simulink model "cobot_dy_create_model"  (R2015b)
settings: Solver=FixedStepAuto  StartTime=0.0  StopTime=10  FixedStep=0.01  RelTol=1e-3
values from neighbouring files (symbols this model uses):
  g = 9.8065    [cobot_gen_traj_and_mass_param.m]    (also in ts2.m; ts3.m)
  ic1 = [ic1xx -ic1xy -ic1xz ... (first row only)    [cobot_gen_traj_and_mass_param.m]
  ic2 = [ic2xx -ic2xy -ic2xz ... (first row only)    [cobot_gen_traj_and_mass_param.m]
  ic3 = [ic3xx -ic3xy -ic3xz ... (first row only)    [cobot_gen_traj_and_mass_param.m]
  ic4 = [ic4xx -ic4xy -ic4xz ... (first row only)    [cobot_gen_traj_and_mass_param.m]
  ic5 = [ic5xx -ic5xy -ic5xz ... (first row only)    [cobot_gen_traj_and_mass_param.m]
  ic6 = [ic6xx -ic6xy -ic6xz ... (first row only)    [cobot_gen_traj_and_mass_param.m]
  m1 = 4.43412756    [cobot_gen_traj_and_mass_param.m]
  m2 = 16.84660904    [cobot_gen_traj_and_mass_param.m]
  m3 = 4.60251258    [cobot_gen_traj_and_mass_param.m]
  m4 = 0.47079045    [cobot_gen_traj_and_mass_param.m]
  m5 = 0.07740646    [cobot_gen_traj_and_mass_param.m]
  m6 = 0.00343612    [cobot_gen_traj_and_mass_param.m]
  P001 = [0 0 d1]'    [cobot_gen_traj_and_mass_param.m]
  P223 = [a3 0 0]'    [cobot_gen_traj_and_mass_param.m]
  P334 = [a4 0 d4]'    [cobot_gen_traj_and_mass_param.m]
  P445 = [0 d5 0]'    [cobot_gen_traj_and_mass_param.m]
  P556 = [0 -d6 0]'    [cobot_gen_traj_and_mass_param.m]
  P667 = [0 0 0]'    [cobot_gen_traj_and_mass_param.m]
  Pc111 = [pc1x pc1y pc1z]'    [cobot_gen_traj_and_mass_param.m]
  Pc222 = [pc2x pc2y pc2z]'    [cobot_gen_traj_and_mass_param.m]
  Pc333 = [pc3x pc3y pc3z]'    [cobot_gen_traj_and_mass_param.m]
  Pc444 = [pc4x pc4y pc4z]'    [cobot_gen_traj_and_mass_param.m]
  Pc555 = [pc5x pc5y pc5z]'    [cobot_gen_traj_and_mass_param.m]
  Pc666 = [pc6x pc6y pc6z]'    [cobot_gen_traj_and_mass_param.m]
libraries: mblibv1 x29
settings Model: Creator=user  LastModifiedBy=12157
settings ConfigComp: CovHTMLOptions=-sRT=1 -sVT=0 -aTS=1 -bRG=1 -bTC=1 -hTR=0 -nFC=0 -nFD=1 -scm=1 -bcm=1 -xEv=0 -xEM=0
settings SimMechanicsCC: VisOnUpdateDiagram=on  VisDuringSimulation=on  LastVizWinPosition=[1 41 1920 938]  CamPosition=[6.48278;4.07346;8.12681;]  CamTarget=[-0.751108;-0.0621973;-0.55549;]  CamUpVector=[-0.477891;-0.569017;0.669208;]  CamHeight=1.40512  VisBackgroundColor=[0.9;0.9;0.95;]  DefaultBodyColor=[1;0;0;]

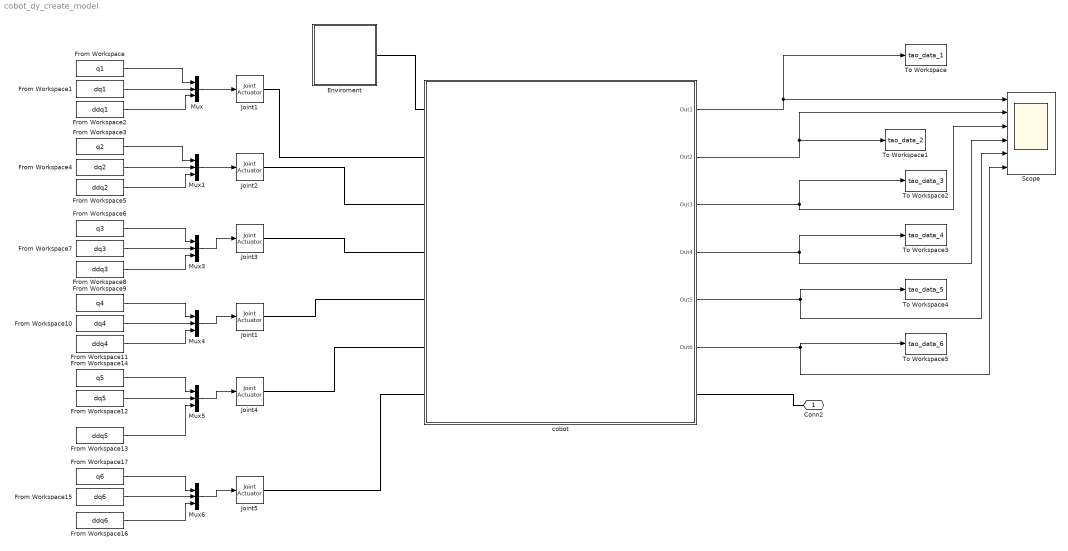
== system cobot_dy_create_model ==
  Enviroment : Subsystem
  From Workspace : FromWorkspace  VariableName=q1  SampleTime=0.01
  From Workspace1 : FromWorkspace  VariableName=dq1  SampleTime=0.01
  From Workspace10 : FromWorkspace  VariableName=dq4  SampleTime=0.01
  From Workspace11 : FromWorkspace  VariableName=ddq4  SampleTime=0.01
  From Workspace12 : FromWorkspace  VariableName=dq5  SampleTime=0.01
  From Workspace13 : FromWorkspace  VariableName=ddq5  SampleTime=0.01
  From Workspace14 : FromWorkspace  VariableName=q5  SampleTime=0.01
  From Workspace15 : FromWorkspace  VariableName=dq6  SampleTime=0.01
  From Workspace16 : FromWorkspace  VariableName=ddq6  SampleTime=0.01
  From Workspace17 : FromWorkspace  VariableName=q6  SampleTime=0.01
  From Workspace2 : FromWorkspace  VariableName=ddq1  SampleTime=0.01
  From Workspace3 : FromWorkspace  VariableName=q2  SampleTime=0.01
  From Workspace4 : FromWorkspace  VariableName=dq2  SampleTime=0.01
  From Workspace5 : FromWorkspace  VariableName=ddq2  SampleTime=0.01
  From Workspace6 : FromWorkspace  VariableName=q3  SampleTime=0.01
  From Workspace7 : FromWorkspace  VariableName=dq3  SampleTime=0.01
  From Workspace8 : FromWorkspace  VariableName=ddq3  SampleTime=0.01
  From Workspace9 : FromWorkspace  VariableName=q4  SampleTime=0.01
  Joint{1,3..5} (4 alike) : mblibv1/Sensors &  Actuators/Joint Actuator  UpdateFromCAD=off  PhysicalDomain=Mechanical  PortType=blob  ActuationStyle=Motion  AngleUnits=deg  ArcVelocityUnits=deg/s  ArcAccelerationUnits=deg/s^2  CoordPositionUnits=m  VelocityUnits=m/s  AccelerationUnits=m/s^2  ForceUnits=N  TorqueUnits=N*m  ActiveIO=on  Width=3  DialogClass=MechanicalActuatorBlock  Primitive=R1  ReferenceFrame=Absolute (World)
  "Joint1 " : mblibv1/Sensors &  Actuators/Joint Actuator  UpdateFromCAD=off  PhysicalDomain=Mechanical  PortType=blob  ActuationStyle=Motion  AngleUnits=deg  ArcVelocityUnits=deg/s  ArcAccelerationUnits=deg/s^2  CoordPositionUnits=m  VelocityUnits=m/s  AccelerationUnits=m/s^2  ForceUnits=N  TorqueUnits=N*m  ActiveIO=on  Width=3  DialogClass=MechanicalActuatorBlock  Primitive=R1  ReferenceFrame=Absolute (World)
  "Joint2 " : mblibv1/Sensors &  Actuators/Joint Actuator  UpdateFromCAD=off  PhysicalDomain=Mechanical  PortType=blob  ActuationStyle=Motion  AngleUnits=deg  ArcVelocityUnits=deg/s  ArcAccelerationUnits=deg/s^2  CoordPositionUnits=m  VelocityUnits=m/s  AccelerationUnits=m/s^2  ForceUnits=N  TorqueUnits=N*m  ActiveIO=on  Width=3  DialogClass=MechanicalActuatorBlock  Primitive=R1  ReferenceFrame=Absolute (World)
  Mux{,1,3..6} (6 alike) : Mux  Inputs=3
  Scope : Scope  NumInputPorts=6
  To Workspace : ToWorkspace  VariableName=tao_data_1  SaveFormat=Timeseries  SampleTime=-1
  To Workspace1 : ToWorkspace  VariableName=tao_data_2  SaveFormat=Timeseries  SampleTime=-1
  To Workspace2 : ToWorkspace  VariableName=tao_data_3  SaveFormat=Timeseries  SampleTime=-1
  To Workspace3 : ToWorkspace  VariableName=tao_data_4  SaveFormat=Timeseries  SampleTime=-1
  To Workspace4 : ToWorkspace  VariableName=tao_data_5  SaveFormat=Timeseries  SampleTime=-1
  To Workspace5 : ToWorkspace  VariableName=tao_data_6  SaveFormat=Timeseries  SampleTime=-1
  cobot : Subsystem
      mask Display: image('cobot.png')
  Conn2 : PMIOPort  Port=1  Side=Left
  wires:
  From Workspace/1 -> Mux/1
  From Workspace1/1 -> Mux/2
  From Workspace2/1 -> Mux/3
  Mux/1 -> "Joint1 "/1
  From Workspace3/1 -> Mux1/1
  From Workspace4/1 -> Mux1/2
  From Workspace5/1 -> Mux1/3
  Mux1/1 -> "Joint2 "/1
  From Workspace6/1 -> Mux3/1
  From Workspace7/1 -> Mux3/2
  From Workspace8/1 -> Mux3/3
  Mux3/1 -> Joint3/1
  From Workspace9/1 -> Mux4/1
  From Workspace10/1 -> Mux4/2
  From Workspace11/1 -> Mux4/3
  Mux4/1 -> Joint1/1
  From Workspace14/1 -> Mux5/1
  From Workspace12/1 -> Mux5/2
  From Workspace13/1 -> Mux5/3
  Mux5/1 -> Joint4/1
  From Workspace17/1 -> Mux6/1
  From Workspace15/1 -> Mux6/2
  From Workspace16/1 -> Mux6/3
  Mux6/1 -> Joint5/1
  cobot/2(Out2) -> Scope/2, To Workspace1/1
  cobot/3(Out3) -> To Workspace2/1, Scope/3
  cobot/4(Out4) -> To Workspace3/1, Scope/4
  cobot/5(Out5) -> Scope/5, To Workspace4/1
  cobot/6(Out6) -> Scope/6, To Workspace5/1
  cobot/1(Out1) -> To Workspace/1, Scope/1
  connections:
  "Joint1 "/RConn1 -- cobot/LConn2
  Conn2/RConn1 -- cobot/RConn1
  Enviroment/RConn1 -- cobot/LConn1
  "Joint2 "/RConn1 -- cobot/LConn3
  Joint3/RConn1 -- cobot/LConn4
  Joint1/RConn1 -- cobot/LConn5
  Joint4/RConn1 -- cobot/LConn6
  Joint5/RConn1 -- cobot/LConn7

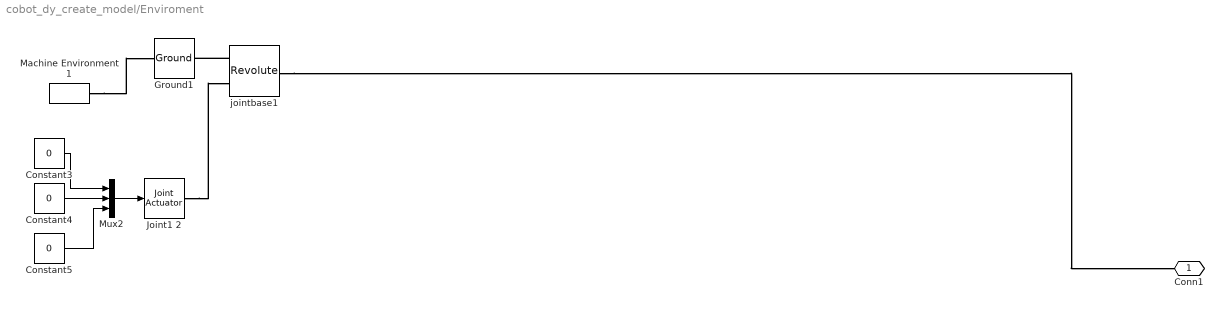
== system cobot_dy_create_model/Enviroment ==
  Constant3 : Constant  Value=0
  Constant4 : Constant  Value=0
  Constant5 : Constant  Value=0
  Ground1 : mblibv1/Bodies/Ground  UpdateFromCAD=off  LeftPortType=env  RightPortType=workingframe  PhysicalDomain=Mechanical  DialogClass=GroundBlock  CoordPosition=[0 0 0]  CoordPositionUnits=m  StateVectorMgrId=0  MachineId=[1 0]  ShowEnvPort=on  ParameterChecksum=[103943624, 4286749661, 2266336483, 2778931322]  TopologyChecksum=[1185680921, 963316717, 888619321, 413900908]
  Joint1 2 : mblibv1/Sensors &  Actuators/Joint Actuator  UpdateFromCAD=off  PhysicalDomain=Mechanical  PortType=blob  ActuationStyle=Motion  AngleUnits=deg  ArcVelocityUnits=deg/s  ArcAccelerationUnits=deg/s^2  CoordPositionUnits=m  VelocityUnits=m/s  AccelerationUnits=m/s^2  ForceUnits=N  TorqueUnits=N*m  ActiveIO=on  Width=3  DialogClass=MechanicalActuatorBlock  Primitive=R1  ReferenceFrame=Absolute (World)
  Machine Environment1 : mblibv1/Bodies/Machine Environment  PortType=env  PhysicalDomain=Mechanical  DialogTemplateClass=MECH.MachineEnvironment  SyncWhenCopied=off  Gravity=[0 0 -g]  GravityUnits=m/s^2  GravityAsSignal=off  Dimensionality=Auto-detect  AnalysisType=Forward dynamics  LinearAssemblyTolerance=1e-3  LinearAssemblyToleranceUnits=m  AngularAssemblyTolerance=1e-3  AngularAssemblyToleranceUnits=rad  ConstraintSolverType=Stabilizing  ConstraintRelTolerance=1e-4  ConstraintAbsTolerance=1e-4  UseRobustSingularityHandling=off  RedundancyAnalysisToleranceType=Automatically select tolerance  RedundancyAnalysisTolerance=1e-14  StatePerturbationType=Fixed  PerturbationSize=1e-5  VisualizeMachine=on  BodyVisualizationType=Use model default body geometries  BodyColorSelMode=Use model default  DefaultBodyColor=[1 0 0]
  Mux2 : Mux  Inputs=3
  jointbase1 : mblibv1/Joints/Revolute  LConnTagsString=__newl0|SA1  RConnTagsString=__newr0  UpdateFromCAD=off  NumSAPorts=1  CutJoint=off  MarkAsCut=off  Primitives=prismatic  PrimitiveProps=R1$World$[0 0 1]$revolute  DialogClass=JointBlock  R1Axis=[0 0 1]
  Conn1 : PMIOPort  Port=1  Side=Right
  wires:
  Constant3/1 -> Mux2/1
  Constant4/1 -> Mux2/2
  Constant5/1 -> Mux2/3
  Mux2/1 -> Joint1 2/1
  connections:
  jointbase1/RConn1 -- Conn1/RConn1
  Joint1 2/RConn1 -- jointbase1/LConn2
  jointbase1/LConn1 -- Ground1/RConn1
  Machine Environment1/RConn1 -- Ground1/LConn1

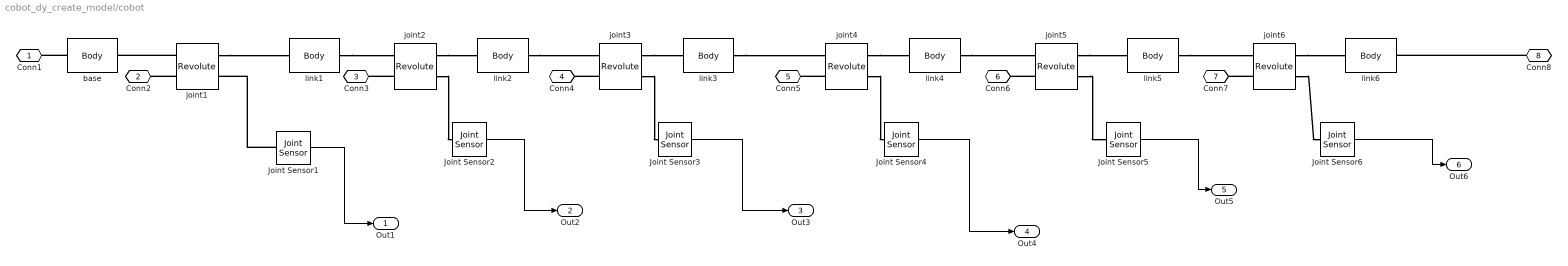
== system cobot_dy_create_model/cobot ==
  Joint Sensor1 : mblibv1/Sensors &  Actuators/Joint Sensor  UpdateFromCAD=off  PhysicalDomain=Mechanical  PortType=blob  Muxed=on  Pose=off  Angle=off  AngleUnits=deg  ArcVelocity=off  ArcVelocityUnits=deg/s  ArcAcceleration=off  ArcAccelerationUnits=deg/s^2  CoordPosition=on  CoordPositionUnits=m  Velocity=off  VelocityUnits=m/s  Acceleration=off  AccelerationUnits=m/s^2  Quaternion=on  QuaternionDT=off  QuaternionDDT=off  QuaternionUnits=off  OutputVector=[1]  ActiveIO=on  Width=1  DialogClass=MechanicalSensorBlock  Primitive=R1  Force=off  ForceUnits=N  Torque=on  TorqueUnits=N*m  ReferenceFrame=Absolute (World)  ReactionSensedSide=Base  ReactionReferenceFrame=Absolute (World)  ReactionForce=off  ReactionForceUnits=N  ReactionMoment=off  ReactionMomentUnits=N*m
  Joint Sensor{2..6} (5 alike) : mblibv1/Sensors &  Actuators/Joint Sensor  UpdateFromCAD=off  PhysicalDomain=Mechanical  PortType=blob  Muxed=off  Pose=off  Angle=off  AngleUnits=deg  ArcVelocity=off  ArcVelocityUnits=deg/s  ArcAcceleration=off  ArcAccelerationUnits=deg/s^2  CoordPosition=on  CoordPositionUnits=m  Velocity=off  VelocityUnits=m/s  Acceleration=off  AccelerationUnits=m/s^2  Quaternion=on  QuaternionDT=off  QuaternionDDT=off  QuaternionUnits=off  OutputVector=[1]  ActiveIO=on  Width=1  DialogClass=MechanicalSensorBlock  Primitive=R1  Force=off  ForceUnits=N  Torque=on  TorqueUnits=N*m  ReferenceFrame=Absolute (World)  ReactionSensedSide=Base  ReactionReferenceFrame=Absolute (World)  ReactionForce=off  ReactionForceUnits=N  ReactionMoment=off  ReactionMomentUnits=N*m
  "base " : mblibv1/Bodies/Body  LConnTagsString=CS1  RConnTagsString=CS2  UpdateFromCAD=off  DialogClass=MechanicalBodyBlock  Mass=1  MassUnits=kg  InertiaUnits=kg*m^2  Inertia=eye(3)  Shape=Cylinder  ShapeDims=[1 1]  ShapeUnits=m  ShapeUse=false  Density=1  DensityUnits=kg/m^3  DensityUse=false  GraphicsMode=MACHINE_DEFAULT  BodyColorSelMode=COLORPALETTE  BodyColor=[1 0 1]  AttachedToCS=CG  CG=Left$CG$P001'*1000/2$CS1$CS1$mm$[0 0 0]$Euler X-Y-Z$deg$CS1$false$none  WorkingFrames=Left$CS1$[0 0 0]$World$World$mm$[0 0 0]$Euler X-Y-Z$deg$WORLD$true$none#Right$CS2$P001'*1000$CS1$CS1$mm$[0 0 0]$Euler X-Y-Z$deg$CS1$true$none  CGPos=P001'*1000/2  CGRot=[0 0 0]  CS0Pos=[]  CS0Rot=[]  CS1Pos=[0 0 0]  CS1Rot=[0 0 0]  CS2Pos=P001'*1000  CS2Rot=[0 0 0]  CS3Pos=[]  CS3Rot=[]  CS4Pos=[]  CS4Rot=[]  CS5Pos=[]  CS5Rot=[]  CS6Pos=[]  CS6Rot=[]  CS7Pos=[]  CS7Rot=[]  CS8Pos=[]  CS8Rot=[]  CS9Pos=[]  CS9Rot=[]  CS10Pos=[]  CS10Rot=[]  CS11Pos=[]  CS11Rot=[]  CS12Pos=[]  CS12Rot=[]  CS13Pos=[]  CS13Rot=[]  CS14Pos=[]  CS14Rot=[]  CS15Pos=[]  CS15Rot=[]  CS16Pos=[]  CS16Rot=[]  CS17Pos=[]  CS17Rot=[]  CS18Pos=[]  CS18Rot=[]  CS19Pos=[]  CS19Rot=[]  CS20Pos=[]  CS20Rot=[]
  joint{1..6} (6 alike) : mblibv1/Joints/Revolute  LConnTagsString=__newl0|SA1  RConnTagsString=__newr0|SA1  UpdateFromCAD=off  NumSAPorts=2  CutJoint=off  MarkAsCut=off  Primitives=prismatic  PrimitiveProps=R1$Base$[0 0 1]$revolute  DialogClass=JointBlock  R1Axis=[0 0 1]
  "link1 " : mblibv1/Bodies/Body  LConnTagsString=CS1  RConnTagsString=CS3  UpdateFromCAD=off  DialogClass=MechanicalBodyBlock  Mass=m1  MassUnits=kg  InertiaUnits=kg*m^2  Inertia=ic1  Shape=Cylinder  ShapeDims=[1 1]  ShapeUnits=m  ShapeUse=false  Density=1  DensityUnits=kg/m^3  DensityUse=false  GraphicsMode=MACHINE_DEFAULT  BodyColorSelMode=COLORPALETTE  BodyColor=[1 1 0]  AttachedToCS=CG  CG=Left$CG$Pc111'*1000$CS1$CS1$mm$[0 0 0]$Euler X-Y-Z$deg$CS1$false$none  WorkingFrames=Left$CS1$[0 0 0]$Adjoining$Adjoining$mm$[0 0 0]$Euler X-Y-Z$deg$Adjoining$true$none#Right$CS2$[0 0 0]$CS1$CS1$mm$[90 0 0]$Euler X-Z-X$deg$CS1$false$none#Right$CS3$[0 0 0]$CS2$CS2$mm$[0 90 0]$Euler X-Z-X$deg$CS2$true$none  CGPos=Pc111'*1000  CGRot=[0 0 0]  CS0Pos=[]  CS0Rot=[]  CS1Pos=[0 0 0]  CS1Rot=[0 0 0]  CS2Pos=[0 0 0]  CS2Rot=[90 0 0]  CS3Pos=[0 0 0]  CS3Rot=[0 90 0]  CS4Pos=[]  CS4Rot=[]  CS5Pos=[]  CS5Rot=[]  CS6Pos=[]  CS6Rot=[]  CS7Pos=[]  CS7Rot=[]  CS8Pos=[]  CS8Rot=[]  CS9Pos=[]  CS9Rot=[]  CS10Pos=[]  CS10Rot=[]  CS11Pos=[]  CS11Rot=[]  CS12Pos=[]  CS12Rot=[]  CS13Pos=[]  CS13Rot=[]  CS14Pos=[]  CS14Rot=[]  CS15Pos=[]  CS15Rot=[]  CS16Pos=[]  CS16Rot=[]  CS17Pos=[]  CS17Rot=[]  CS18Pos=[]  CS18Rot=[]  CS19Pos=[]  CS19Rot=[]  CS20Pos=[]  CS20Rot=[]
  link2 : mblibv1/Bodies/Body  LConnTagsString=CS1  RConnTagsString=CS2  UpdateFromCAD=off  DialogClass=MechanicalBodyBlock  Mass=m2  MassUnits=kg  InertiaUnits=kg*m^2  Inertia=ic2  Shape=Cylinder  ShapeDims=[1 1]  ShapeUnits=m  ShapeUse=false  Density=1  DensityUnits=kg/m^3  DensityUse=false  GraphicsMode=MACHINE_DEFAULT  BodyColorSelMode=COLORPALETTE  BodyColor=[0.23137 0.44314 0.33726]  AttachedToCS=CG  CG=Left$CG$Pc222'*1000$CS1$CS1$mm$[0 0 0]$Euler X-Y-Z$deg$CS1$false$none  WorkingFrames=Left$CS1$[0 0 0]$Adjoining$Adjoining$mm$[0 0 0]$Euler X-Y-Z$deg$Adjoining$true$none#Right$CS2$P223*1000$CS1$CS1$mm$[0 0 -90]$Euler X-Y-Z$deg$CS1$true$none  CGPos=Pc222'*1000  CGRot=[0 0 0]  CS0Pos=[]  CS0Rot=[]  CS1Pos=[0 0 0]  CS1Rot=[0 0 0]  CS2Pos=P223*1000  CS2Rot=[0 0 -90]  CS3Pos=[]  CS3Rot=[]  CS4Pos=[]  CS4Rot=[]  CS5Pos=[]  CS5Rot=[]  CS6Pos=[]  CS6Rot=[]  CS7Pos=[]  CS7Rot=[]  CS8Pos=[]  CS8Rot=[]  CS9Pos=[]  CS9Rot=[]  CS10Pos=[]  CS10Rot=[]  CS11Pos=[]  CS11Rot=[]  CS12Pos=[]  CS12Rot=[]  CS13Pos=[]  CS13Rot=[]  CS14Pos=[]  CS14Rot=[]  CS15Pos=[]  CS15Rot=[]  CS16Pos=[]  CS16Rot=[]  CS17Pos=[]  CS17Rot=[]  CS18Pos=[]  CS18Rot=[]  CS19Pos=[]  CS19Rot=[]  CS20Pos=[]  CS20Rot=[]
  link3 : mblibv1/Bodies/Body  LConnTagsString=CS1  RConnTagsString=CS2  UpdateFromCAD=off  DialogClass=MechanicalBodyBlock  Mass=m3  MassUnits=kg  InertiaUnits=kg*m^2  Inertia=ic3  Shape=Cylinder  ShapeDims=[1 1]  ShapeUnits=m  ShapeUse=false  Density=1  DensityUnits=kg/m^3  DensityUse=false  GraphicsMode=MACHINE_DEFAULT  BodyColorSelMode=COLORPALETTE  BodyColor=[1 0 0]  AttachedToCS=CG  CG=Left$CG$Pc333'*1000$CS1$CS1$mm$[0 0 0]$Euler X-Y-Z$deg$CS1$false$none  WorkingFrames=Left$CS1$[0 0 0]$Adjoining$Adjoining$mm$[0 0 0]$Euler X-Y-Z$deg$Adjoining$true$none#Right$CS2$P334'*1000$CS1$CS1$mm$[0 0 0]$Euler X-Y-Z$deg$CS1$true$none  CGPos=Pc333'*1000  CGRot=[0 0 0]  CS0Pos=[]  CS0Rot=[]  CS1Pos=[0 0 0]  CS1Rot=[0 0 0]  CS2Pos=P334'*1000  CS2Rot=[0 0 0]  CS3Pos=[]  CS3Rot=[]  CS4Pos=[]  CS4Rot=[]  CS5Pos=[]  CS5Rot=[]  CS6Pos=[]  CS6Rot=[]  CS7Pos=[]  CS7Rot=[]  CS8Pos=[]  CS8Rot=[]  CS9Pos=[]  CS9Rot=[]  CS10Pos=[]  CS10Rot=[]  CS11Pos=[]  CS11Rot=[]  CS12Pos=[]  CS12Rot=[]  CS13Pos=[]  CS13Rot=[]  CS14Pos=[]  CS14Rot=[]  CS15Pos=[]  CS15Rot=[]  CS16Pos=[]  CS16Rot=[]  CS17Pos=[]  CS17Rot=[]  CS18Pos=[]  CS18Rot=[]  CS19Pos=[]  CS19Rot=[]  CS20Pos=[]  CS20Rot=[]
  link4 : mblibv1/Bodies/Body  LConnTagsString=CS1  RConnTagsString=CS2  UpdateFromCAD=off  DialogClass=MechanicalBodyBlock  Mass=m4  MassUnits=kg  InertiaUnits=kg*m^2  Inertia=ic4  Shape=Cylinder  ShapeDims=[1 1]  ShapeUnits=m  ShapeUse=false  Density=1  DensityUnits=kg/m^3  DensityUse=false  GraphicsMode=MACHINE_DEFAULT  BodyColorSelMode=COLORPALETTE  BodyColor=[0.6 0.2 0]  AttachedToCS=CG  CG=Left$CG$Pc444'*1000$CS1$CS1$mm$[0 0 0]$Euler X-Y-Z$deg$CS1$false$none  WorkingFrames=Left$CS1$[0 0 0]$Adjoining$Adjoining$mm$[0 0 0]$Euler X-Y-Z$deg$Adjoining$true$none#Right$CS2$P445'*1000$CS1$CS1$mm$[-90 0 90]$Euler X-Y-Z$deg$CS1$true$none  CGPos=Pc444'*1000  CGRot=[0 0 0]  CS0Pos=[]  CS0Rot=[]  CS1Pos=[0 0 0]  CS1Rot=[0 0 0]  CS2Pos=P445'*1000  CS2Rot=[-90 0 90]  CS3Pos=[]  CS3Rot=[]  CS4Pos=[]  CS4Rot=[]  CS5Pos=[]  CS5Rot=[]  CS6Pos=[]  CS6Rot=[]  CS7Pos=[]  CS7Rot=[]  CS8Pos=[]  CS8Rot=[]  CS9Pos=[]  CS9Rot=[]  CS10Pos=[]  CS10Rot=[]  CS11Pos=[]  CS11Rot=[]  CS12Pos=[]  CS12Rot=[]  CS13Pos=[]  CS13Rot=[]  CS14Pos=[]  CS14Rot=[]  CS15Pos=[]  CS15Rot=[]  CS16Pos=[]  CS16Rot=[]  CS17Pos=[]  CS17Rot=[]  CS18Pos=[]  CS18Rot=[]  CS19Pos=[]  CS19Rot=[]  CS20Pos=[]  CS20Rot=[]
  link5 : mblibv1/Bodies/Body  LConnTagsString=CS1  RConnTagsString=CS2  UpdateFromCAD=off  DialogClass=MechanicalBodyBlock  Mass=m5  MassUnits=kg  InertiaUnits=kg*m^2  Inertia=ic5  Shape=Cylinder  ShapeDims=[1 1]  ShapeUnits=m  ShapeUse=false  Density=1  DensityUnits=kg/m^3  DensityUse=false  GraphicsMode=MACHINE_DEFAULT  BodyColorSelMode=COLORPALETTE  BodyColor=[1 0 0]  AttachedToCS=CG  CG=Left$CG$Pc555'*1000$CS1$CS1$mm$[0 0 0]$Euler X-Y-Z$deg$CS1$false$none  WorkingFrames=Left$CS1$[0 0 0]$Adjoining$Adjoining$mm$[0 0 0]$Euler X-Y-Z$deg$Adjoining$true$none#Right$CS2$P556'*1000$CS1$CS1$mm$[90 0 180]$Euler X-Y-Z$deg$CS1$true$none  CGPos=Pc555'*1000  CGRot=[0 0 0]  CS0Pos=[]  CS0Rot=[]  CS1Pos=[0 0 0]  CS1Rot=[0 0 0]  CS2Pos=P556'*1000  CS2Rot=[90 0 180]  CS3Pos=[]  CS3Rot=[]  CS4Pos=[]  CS4Rot=[]  CS5Pos=[]  CS5Rot=[]  CS6Pos=[]  CS6Rot=[]  CS7Pos=[]  CS7Rot=[]  CS8Pos=[]  CS8Rot=[]  CS9Pos=[]  CS9Rot=[]  CS10Pos=[]  CS10Rot=[]  CS11Pos=[]  CS11Rot=[]  CS12Pos=[]  CS12Rot=[]  CS13Pos=[]  CS13Rot=[]  CS14Pos=[]  CS14Rot=[]  CS15Pos=[]  CS15Rot=[]  CS16Pos=[]  CS16Rot=[]  CS17Pos=[]  CS17Rot=[]  CS18Pos=[]  CS18Rot=[]  CS19Pos=[]  CS19Rot=[]  CS20Pos=[]  CS20Rot=[]
  link6 : mblibv1/Bodies/Body  LConnTagsString=CS1  RConnTagsString=CS2  UpdateFromCAD=off  DialogClass=MechanicalBodyBlock  Mass=m6  MassUnits=kg  InertiaUnits=kg*m^2  Inertia=ic6  Shape=Cylinder  ShapeDims=[1 1]  ShapeUnits=m  ShapeUse=false  Density=1  DensityUnits=kg/m^3  DensityUse=false  GraphicsMode=MACHINE_DEFAULT  GraphicsFileName=.\model\RobotPart6.STL  BodyColorSelMode=COLORPALETTE  BodyColor=[1 0 0]  AttachedToCS=CG  CG=Left$CG$Pc666'*1000$CS1$CS1$mm$[0 0 0]$Euler X-Y-Z$deg$CS1$false$none  WorkingFrames=Left$CS1$[0 0 0]$Adjoining$Adjoining$mm$[0 0 0]$Euler X-Y-Z$deg$Adjoining$true$none#Right$CS2$P667'*1000$CS1$CS1$mm$[0 0 0]$Euler X-Y-Z$deg$CS1$true$none  CGPos=Pc666'*1000  CGRot=[0 0 0]  CS0Pos=[]  CS0Rot=[]  CS1Pos=[0 0 0]  CS1Rot=[0 0 0]  CS2Pos=P667'*1000  CS2Rot=[0 0 0]  CS3Pos=[]  CS3Rot=[]  CS4Pos=[]  CS4Rot=[]  CS5Pos=[]  CS5Rot=[]  CS6Pos=[]  CS6Rot=[]  CS7Pos=[]  CS7Rot=[]  CS8Pos=[]  CS8Rot=[]  CS9Pos=[]  CS9Rot=[]  CS10Pos=[]  CS10Rot=[]  CS11Pos=[]  CS11Rot=[]  CS12Pos=[]  CS12Rot=[]  CS13Pos=[]  CS13Rot=[]  CS14Pos=[]  CS14Rot=[]  CS15Pos=[]  CS15Rot=[]  CS16Pos=[]  CS16Rot=[]  CS17Pos=[]  CS17Rot=[]  CS18Pos=[]  CS18Rot=[]  CS19Pos=[]  CS19Rot=[]  CS20Pos=[]  CS20Rot=[]
  Conn1 : PMIOPort  Port=1  Side=Left
  Conn2 : PMIOPort  Port=2  Side=Left
  Conn3 : PMIOPort  Port=3  Side=Left
  Conn4 : PMIOPort  Port=4  Side=Left
  Conn5 : PMIOPort  Port=5  Side=Left
  Conn6 : PMIOPort  Port=6  Side=Left
  Conn7 : PMIOPort  Port=7  Side=Left
  Conn8 : PMIOPort  Port=8  Side=Right
  Out1 : Outport
  Out2 : Outport  Port=2
  Out3 : Outport  Port=3
  Out4 : Outport  Port=4
  Out5 : Outport  Port=5
  Out6 : Outport  Port=6
  wires:
  Joint Sensor3/1 -> Out3/1
  Joint Sensor4/1 -> Out4/1
  Joint Sensor1/1 -> Out1/1
  Joint Sensor6/1 -> Out6/1
  Joint Sensor2/1 -> Out2/1
  Joint Sensor5/1 -> Out5/1
  connections:
  joint6/RConn2 -- Joint Sensor6/LConn1
  joint6/RConn1 -- link6/LConn1
  joint5/RConn1 -- link5/LConn1
  joint5/RConn2 -- Joint Sensor5/LConn1
  joint1/RConn1 -- "link1 "/LConn1
  Joint Sensor1/LConn1 -- joint1/RConn2
  "base "/LConn1 -- Conn1/RConn1
  joint4/LConn2 -- Conn5/RConn1
  joint6/LConn2 -- Conn7/RConn1
  joint2/RConn2 -- Joint Sensor2/LConn1
  "link1 "/RConn1 -- joint2/LConn1
  joint2/RConn1 -- link2/LConn1
  joint4/RConn2 -- Joint Sensor4/LConn1
  joint4/RConn1 -- link4/LConn1
  link5/RConn1 -- joint6/LConn1
  Conn8/RConn1 -- link6/RConn1
  link2/RConn1 -- joint3/LConn1
  joint3/RConn1 -- link3/LConn1
  joint3/RConn2 -- Joint Sensor3/LConn1
  joint1/LConn2 -- Conn2/RConn1
  joint5/LConn2 -- Conn6/RConn1
  joint3/LConn2 -- Conn4/RConn1
  joint2/LConn2 -- Conn3/RConn1
  link3/RConn1 -- joint4/LConn1
  link4/RConn1 -- joint5/LConn1
  joint1/LConn1 -- "base "/RConn1
